simulink model "electro_mechanical_model"  (R2022a)
settings: Solver=VariableStepAuto  StartTime=0.0  StopTime=10000  RelTol=1e-3
values from neighbouring files (symbols this model uses):
  Ts = 5E-6    (= 5e-06)    [motor_variables.m]
undefined symbols (not defined in the file or in its folder): sigbuilder_block
libraries: fl_lib x42, nesl_utility x17, ee_lib x5, sdl_lib x2
settings Model: Creator=OADEBAJO  LastModifiedBy=oadebajo

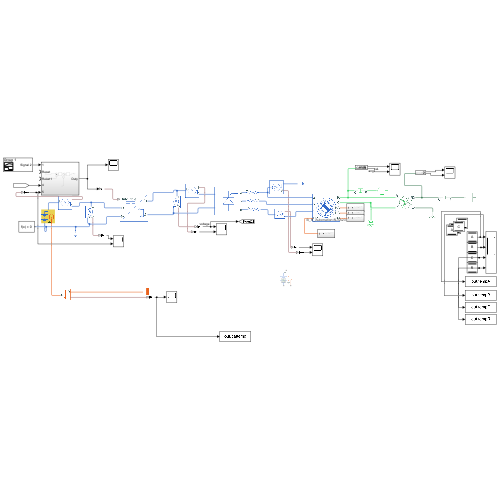
[thumbnail: Simulink's stored preview of the top-level diagram]
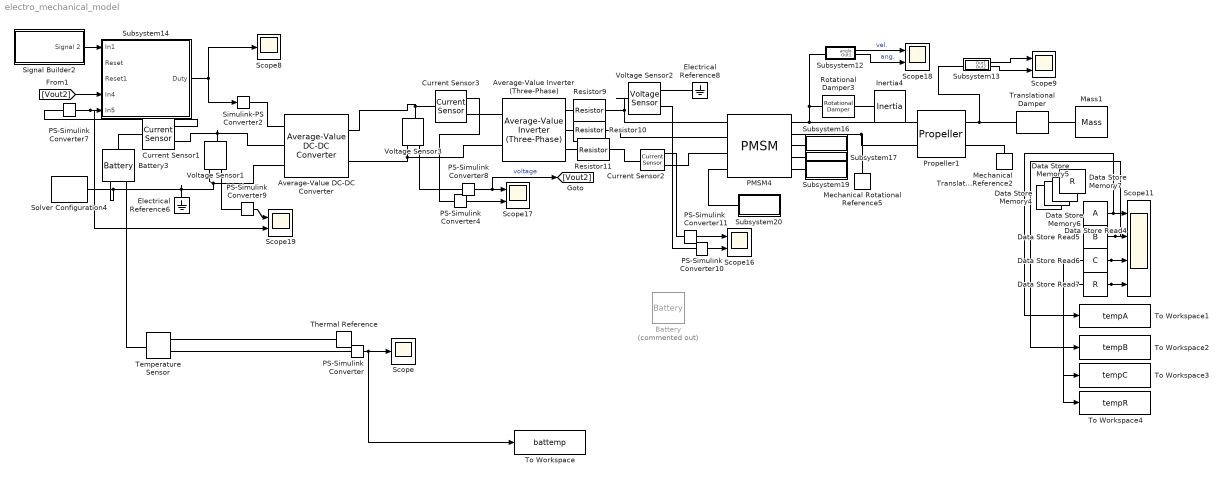
== system electro_mechanical_model ==
  Average-Value Inverter (Three-Phase) : ee_lib/Semiconductors & Converters/Converters/Average-Value Inverter (Three-Phase)  port_option=ee.enum.threePhasePort.expanded  FRated=60 Hz  PhaseShift=60 deg  voltage_ratio=sqrt(6) / pi  Pfixed=1e3 W  v_on=100 V  v_off=75 V
      settings: SourceProductBaseCode=PS  InternalSimscapePortConfiguration="{\"Bottom\":[],\"Left\":[{\"id\":\"p\",\"label\":\"+\",\"type\":\"foundation.electrical.electrical\"},{\"id\":\"n\",\"label\":\"-\",\"type\":\"foundation.electrical.electrical\"}],\"Right\":[{\"id\":\"a\",\"label\":\"a\",\"type\":\"foundation.electrical.electrical\"},{\"id\":\"b\",\"label\":\"b\",\"type\":\"foundation.electrical.electrical\"},{\"id\":\"c\",\"label\":\"c\",\"type\":\"foundation.electrical.electrical\"}],\"Top\":[]}"
  Average-Value DC-DC Converter : ee_lib/Semiconductors & Converters/Converters/Average-Value DC-DC Converter  control_option=ee.enum.converters.controlinput.dutycycle  converter_type=ee.enum.converters.dcdctype.buckboost  efficiency_option=ee.enum.converters.efficiency.constant  efficiency_fixed=100  i_vec=[0, 2, 5] A  efficiency_vec=[90, 95, 98]
      settings: SourceProductBaseCode=PS  InternalSimscapePortConfiguration="{\"Bottom\":[],\"Left\":[{\"id\":\"DutyCycle\",\"label\":\"DutyCycle\",\"type\":\"input\"},{\"id\":\"p1\",\"label\":\"1+\",\"type\":\"foundation.electrical.electrical\"},{\"id\":\"n1\",\"label\":\"1-\",\"type\":\"foundation.electrical.electrical\"}],\"Right\":[{\"id\":\"p2\",\"label\":\"2+\",\"type\":\"foundation.electrical.electrical\"},{\"id\":\"n2\",\"label\":\"2-\",\"type\":\"foundation.electrical.electrical\"}],\"Top\":[]}"
  Battery : ee_lib/Sources/Battery  Commented=on  Vnom=300 V  prm_dir=ee.enum.batterybasic.prm_dir.disabled  R1_dis=2 Ohm  R1_ch=2 Ohm  R1=0.001 Ohm  prm_AH=ee.enum.batterybasic.prm_AH.infinite  AH=50 A*hr  V1=11.5 V  AH1=25 A*hr  prm_R2=ee.enum.batterybasic.prm_R2.disabled  R2=2000 Ohm  prm_dyn=ee.enum.batterybasic.prm_dyn.off  Rp1=0.005 Ohm  tau1=30 s  Rp2=0.005 Ohm  tau2=30 s  Rp3=0.005 Ohm  tau3=30 s  Rp4=0.005 Ohm  tau4=30 s  Rp5=0.005 Ohm  tau5=30 s  prm_fade=ee.enum.batterybasic.prm_fade.disabled  N_fade=100  AH_fade=45 A*hr  R1_fade=2.02 Ohm  R1_ch_fade=2.02 Ohm  V1_fade=10.35 V  prm_age=ee.enum.batterybasic.prm_age.disabled  prm_age_OCV=ee.enum.batterybasic.prm_age_OCV.OCV  OCV_age=0.9  SOC_age=60  delta_time_age_vec=[0] d  temperature_age_vec=[273] K  OCV_scaling_age=2.2134e6  OCV_offset_age=1.632e6  temp_exp_age=0.515833569 V  t_exp_age=0.75  i_specify=off  i_priority=None  i=0 A  i_nominal_specify=off  i_nominal_unit=A  i_nominal_value=1  v_specify=off  v_priority=None  v=0 V  v_nominal_specify=off  v_nominal_unit=V  v_nominal_value=1  charge_specify=off  charge_priority=High  charge=50 A*hr  charge_nominal_specify=off  charge_nominal_unit=A*hr  charge_nominal_value=1  num_cycles_specify=off  num_cycles_priority=High  num_cycles=0  num_cycles_nominal_specify=off  num_cycles_nominal_unit=1  num_cycles_nominal_value=1  Tmeas=298.15 K  Tmeas_age=298.15 K  Vnom_T2=12 V  R1_T2=2.2 Ohm  R1_T2_dis=2.2 Ohm  R1_T2_ch=2.2 Ohm  V1_T2=11.4 V  R2_T2=2200 Ohm  Rp1_T2=0.005 Ohm  tau1_T2=30 s  Rp2_T2=0.005 Ohm  tau2_T2=30 s  Rp3_T2=0.005 Ohm  tau3_T2=30 s  Rp4_T2=0.005 Ohm  tau4_T2=30 s  Rp5_T2=0.005 Ohm  tau5_T2=30 s  Tmeas2=273.15 K  thermal_mass=30000 J/K  temperature_specify=off  temperature_priority=High  temperature=298.15 K  temperature_nominal_specify=off  temperature_nominal_unit=K  temperature_nominal_value=1
      settings: InternalSimscapePortConfiguration="{\"Bottom\":[],\"Left\":[{\"id\":\"p\",\"label\":\"+\",\"type\":\"foundation.electrical.electrical\"}],\"Right\":[{\"id\":\"n\",\"label\":\"-\",\"type\":\"foundation.electrical.electrical\"},{\"id\":\"H\",\"label\":\"H\",\"type\":\"foundation.thermal.thermal\"}],\"Top\":[]}"
  Battery3 : ee_lib/Sources/Battery  Vnom=300 V  prm_dir=ee.enum.batterybasic.prm_dir.disabled  R1_dis=2 Ohm  R1_ch=2 Ohm  R1=0.001 Ohm  prm_AH=ee.enum.batterybasic.prm_AH.infinite  AH=50 A*hr  V1=11.5 V  AH1=25 A*hr  prm_R2=ee.enum.batterybasic.prm_R2.disabled  R2=2000 Ohm  prm_dyn=ee.enum.batterybasic.prm_dyn.off  Rp1=0.005 Ohm  tau1=30 s  Rp2=0.005 Ohm  tau2=30 s  Rp3=0.005 Ohm  tau3=30 s  Rp4=0.005 Ohm  tau4=30 s  Rp5=0.005 Ohm  tau5=30 s  prm_fade=ee.enum.batterybasic.prm_fade.disabled  N_fade=100  AH_fade=45 A*hr  R1_fade=2.02 Ohm  R1_ch_fade=2.02 Ohm  V1_fade=10.35 V  prm_age=ee.enum.batterybasic.prm_age.disabled  prm_age_OCV=ee.enum.batterybasic.prm_age_OCV.OCV  OCV_age=0.9  SOC_age=60  delta_time_age_vec=[0] d  temperature_age_vec=[273] K  OCV_scaling_age=2.2134e6  OCV_offset_age=1.632e6  temp_exp_age=0.515833569 V  t_exp_age=0.75  i_specify=off  i_priority=None  i=0 A  i_nominal_specify=off  i_nominal_unit=A  i_nominal_value=1  v_specify=off  v_priority=None  v=0 V  v_nominal_specify=off  v_nominal_unit=V  v_nominal_value=1  charge_specify=off  charge_priority=High  charge=50 A*hr  charge_nominal_specify=off  charge_nominal_unit=A*hr  charge_nominal_value=1  num_cycles_specify=off  num_cycles_priority=High  num_cycles=0  num_cycles_nominal_specify=off  num_cycles_nominal_unit=1  num_cycles_nominal_value=1  Tmeas=298.15 K  Tmeas_age=298.15 K  Vnom_T2=300 V  R1_T2=0.01 Ohm  R1_T2_dis=2.2 Ohm  R1_T2_ch=2.2 Ohm  V1_T2=11.4 V  R2_T2=2200 Ohm  Rp1_T2=0.005 Ohm  tau1_T2=30 s  Rp2_T2=0.005 Ohm  tau2_T2=30 s  Rp3_T2=0.005 Ohm  tau3_T2=30 s  Rp4_T2=0.005 Ohm  tau4_T2=30 s  Rp5_T2=0.005 Ohm  tau5_T2=30 s  Tmeas2=273.15 K  thermal_mass=30000 J/K  temperature_specify=off  temperature_priority=High  temperature=298.15 K  temperature_nominal_specify=off  temperature_nominal_unit=K  temperature_nominal_value=1
      settings: InternalSimscapePortConfiguration="{\"Bottom\":[],\"Left\":[{\"id\":\"p\",\"label\":\"+\",\"type\":\"foundation.electrical.electrical\"}],\"Right\":[{\"id\":\"n\",\"label\":\"-\",\"type\":\"foundation.electrical.electrical\"},{\"id\":\"H\",\"label\":\"H\",\"type\":\"foundation.thermal.thermal\"}],\"Top\":[]}"
  Current Sensor1 : fl_lib/Electrical/Electrical Sensors/Current Sensor
      settings: SourceProductBaseCode=PW,SS,VE
  Current Sensor2 : fl_lib/Electrical/Electrical Sensors/Current Sensor
      settings: SourceProductBaseCode=PW,SS,VE
  Current Sensor3 : fl_lib/Electrical/Electrical Sensors/Current Sensor
      settings: SourceProductBaseCode=PW,SS,VE
  Data Store Memory4 : DataStoreMemory  WriteAfterWriteMsg=warning  ShowAdditionalParam=off
  Data Store Memory5 : DataStoreMemory  DataStoreName=B  WriteAfterWriteMsg=warning  ShowAdditionalParam=off
  Data Store Memory6 : DataStoreMemory  DataStoreName=C  WriteAfterWriteMsg=warning  ShowAdditionalParam=off
  Data Store Memory7 : DataStoreMemory  DataStoreName=R  WriteAfterWriteMsg=warning  ShowAdditionalParam=off
  Data Store Read4 : DataStoreRead  IndexOptions=Index vector (dialog)  Indices=1  OutputSizes=1
  Data Store Read5 : DataStoreRead  DataStoreName=B  IndexOptions=Index vector (dialog)  Indices=1  OutputSizes=1
  Data Store Read6 : DataStoreRead  DataStoreName=C  IndexOptions=Index vector (dialog)  Indices=1  OutputSizes=1
  Data Store Read7 : DataStoreRead  DataStoreName=R  IndexOptions=Index vector (dialog)  Indices=1  OutputSizes=1
  Electrical Reference6 : fl_lib/Electrical/Electrical Elements/Electrical Reference
      settings: SourceProductBaseCode=PW,SS,VE
  Electrical Reference8 : fl_lib/Electrical/Electrical Elements/Electrical Reference
      settings: SourceProductBaseCode=PW,SS,VE
  Inertia4 : fl_lib/Mechanical/Rotational Elements/Inertia  inertia=0.01 kg*m^2  num_ports=foundation.enum.numPorts2.one  w_specify=off  w_priority=High  w=0 rad/s  w_nominal_specify=off  w_nominal_unit=rad/s  w_nominal_value=1  t_specify=off  t_priority=None  t=0 N*m  t_nominal_specify=off  t_nominal_unit=N*m  t_nominal_value=1
      settings: SourceProductBaseCode=PW,SS,VE
  Mass1 : fl_lib/Mechanical/Translational Elements/Mass  mass=1 kg  num_ports=foundation.enum.numPorts2.one  v_specify=off  v_priority=High  v=0 m/s  v_nominal_specify=off  v_nominal_unit=m/s  v_nominal_value=1  f_specify=off  f_priority=None  f=0 N  f_nominal_specify=off  f_nominal_unit=N  f_nominal_value=1
      settings: SourceProductBaseCode=PW,SS,VE
  Mechanical Rotational Reference5 : fl_lib/Mechanical/Rotational Elements/Mechanical Rotational Reference
      settings: SourceProductBaseCode=PW,SS,VE
  Mechanical Translational Reference2 : fl_lib/Mechanical/Translational Elements/Mechanical Translational Reference
      settings: SourceProductBaseCode=PW,SS,VE
  PMSM4 : ee_lib/Electromechanical/Permanent Magnet/PMSM  Tag={'toolbox/physmod/elec/library/m/ee_lib_parts';'Electromechanical/Permanent_Magnet/PMSM/B_R_Automation/x8LSA23.xml'}  port_option=ee.enum.threePhasePort.expanded  winding_type=ee.enum.statorconnection.wye  machine_param=ee.enum.pmsm.parameterization.constant  nPolePairs=2  pmflux_param=ee.enum.pmflux.fluxlinkage  pm_flux_linkage=0.171455326591285 Wb  torque_constant=0.342910653182571 N*m/A  back_emf_constant=0.342910653182571 V/(rad/s)  stator_param=ee.enum.statorparam.LdLqL0  Ld=0.0825 H  Lq=0.0825 H  idVec=[-200 0 200] % Parameter not set A  iqVec=[-200 0 200] % Parameter not set A  LdMatrix=[0.0002 0.0002 0.0002;0.0002 0.0002 0.0002;0.0002 0.0002 0.0002] % Parameter not set H  LqMatrix=[0.0002 0.0002 0.0002;0.0002 0.0002 0.0002;0.0002 0.0002 0.0002] % Parameter not set H  PmMatrix=[0.1 0.1 0.1;0.1 0.1 0.1;0.1 0.1 0.1] Wb  ktMatrix=[0.18 0.18 0.18;0.18 0.18 0.18;0.18 0.18 0.18] N*m/A  keMatrix=[0.18 0.18 0.18;0.18 0.18 0.18;0.18 0.18 0.18] % Parameter not set V/(rad/s)  L0=[] % Parameter not set H  Ls=0.0002 H  Lm=-2e-05 H  Ms=2e-05 H  Rs=84 Ohm  zero_sequence=ee.enum.park.zerosequence.exclude  axes_param=ee.enum.rotorangle.daxis  loss_param=ee.enum.ironloss.none  losses_oc=[0 0 0] % Parameter not set W  losses_sc=[0 0 0] % Parameter not set W  f_losses=60 % Parameter not set Hz  Isc_losses=95 % Parameter not set A  J=7e-06 kg*m^2  lam=0 % Parameter not set N*m/(rad/s)  i_d_specify=off  i_d_priority=None  i_d=0 A  i_d_nominal_specify=off  i_d_nominal_unit=A  i_d_nominal_value=1  i_q_specify=off  i_q_priority=None  i_q=0 A  i_q_nominal_specify=off  i_q_nominal_unit=A  i_q_nominal_value=1  torque_specify=off  torque_priority=None  torque=0 N*m  torque_nominal_specify=off  torque_nominal_unit=N*m  torque_nominal_value=1  angular_velocity_specify=off  angular_velocity_priority=High  angular_velocity=0 rpm  angular_velocity_nominal_specify=off  angular_velocity_nominal_unit=rpm  angular_velocity_nominal_value=1  angular_position_specify=off  angular_position_priority=High  angular_position=0 deg  angular_position_nominal_specify=off  angular_position_nominal_unit=deg  angular_position_nominal_value=1  alpha=0.00393 % Parameter not set 1/K  alpha_flux=-0.001 % Parameter not set 1/K  Tmeas=298.15 % Parameter not set K  stator_thermal_mass=100 % Parameter not set J/K  rotor_thermal_mass=200 % Parameter not set J/K  Rm_percent_rotor=90  Rd_percent_rotor=30  temperatureA_specify=on  temperatureA_priority=None  temperatureA=25 degC  temperatureA_nominal_specify=off  temperatureA_nominal_unit=degC  temperatureA_nominal_value=1  temperatureB_specify=on  temperatureB_priority=None  temperatureB=25 degC  temperatureB_nominal_specify=off  temperatureB_nominal_unit=degC  temperatureB_nominal_value=1  temperatureC_specify=on  temperatureC_priority=None  temperatureC=25 degC  temperatureC_nominal_specify=off  temperatureC_nominal_unit=degC  temperatureC_nominal_value=1  temperatureR_specify=on  temperatureR_priority=None  temperatureR=25 degC  temperatureR_nominal_specify=off  temperatureR_nominal_unit=degC  temperatureR_nominal_value=1
      settings: AttributesFormatString=B_R_Automation:8LSA23  InternalSimscapePortConfiguration="{\"Bottom\":[],\"Left\":[{\"id\":\"a\",\"label\":\"a\",\"type\":\"foundation.electrical.electrical\"},{\"id\":\"b\",\"label\":\"b\",\"type\":\"foundation.electrical.electrical\"},{\"id\":\"c\",\"label\":\"c\",\"type\":\"foundation.electrical.electrical\"},{\"id\":\"HR\",\"label\":\"HR\",\"type\":\"foundation.thermal.thermal\"}],\"Right\":[{\"id\":\"R\",\"label\":\"R\",\"type\":\"foundation.mechanical.rotational.rotational\"},{\"id\":\"C\",\"label\":\"C\",\"type\":\"foundation.mechanical.rotational.rotational\"},{\"id\":\"HA\",\"label\":\"HA\",\"type\":\"foundation.thermal.thermal\"},{\"id\":\"HB\",\"label\":\"HB\",\"type\":\"foundation.thermal.thermal\"},{\"id\":\"HC\",\"label\":\"HC\",\"type\":\"foundation.thermal.thermal\"}],\"Top\":[]}"
  PS-Simulink Converter{,4,10..11} (4 alike) : nesl_utility/PS-Simulink Converter  PhysicalDomain=network_engine_domain  SubClassName=ps_output  LeftPortType=input  RightPortType=output  PseudoPeriodic=off  Frequencies=[]  VectorFormat=inherit  Unit=inherit  AffineConversion=off
      settings: SourceProductBaseCode=SS,PW,VE
  PS-Simulink Converter7 : nesl_utility/PS-Simulink Converter  PhysicalDomain=network_engine_domain  SubClassName=ps_output  LeftPortType=input  RightPortType=output  PseudoPeriodic=off  Frequencies=[]  VectorFormat=1-D array  Unit=A  AffineConversion=off
      settings: SourceProductBaseCode=SS,PW,VE
  PS-Simulink Converter8 : nesl_utility/PS-Simulink Converter  PhysicalDomain=network_engine_domain  SubClassName=ps_output  LeftPortType=input  RightPortType=output  PseudoPeriodic=off  Frequencies=[]  VectorFormat=1-D array  Unit=V  AffineConversion=off
      settings: SourceProductBaseCode=SS,PW,VE
  PS-Simulink Converter9 : nesl_utility/PS-Simulink Converter  PhysicalDomain=network_engine_domain  SubClassName=ps_output  LeftPortType=input  RightPortType=output  PseudoPeriodic=off  Frequencies=[]  VectorFormat=1-D array  Unit=V  AffineConversion=off
      settings: SourceProductBaseCode=SS,PW,VE
  Propeller1 : sdl_lib/Engines & Motors/Propeller  parameterization=sdl.enum.PropellerParameterization.Constant  pitch_type=foundation.enum.constant_controlled.constant  D=0.2 m  kt_const=0.25  kq_const=0.05  kt_poly_fixed=[.063, -.19, -.25, .37]  kq_poly_fixed=[.0043, -.021, -.03, .05]  pitch_ratio_TLU=[-.5, .5, .7, .9, 1.1, 1.4]  kt_poly_TLU=[.04, -.1, -.24, .12; .118, -.24, -.24, .19; .082, -.21, -.25, .28; .063, -.19, -.25, .37; .055, -.17, -.25, .45; .064, -.21, -.19, .55]  kq_poly_TLU=[.02, -.06, -.02, .02; .04, -.034, -.016, .018; .0076, -.02, -.023, .031; .0043, -.021, -.03, .05; .0047, -.024, -.036, .073; .0045, -.025, -.044, .11]  J_tab_TLU=[0, .3, .5, .7, .9, 1.2, 1.5]  kt_tab_fixed=[.37, .28, .21, .12, .033, -.098, -.23]  kq_tab_fixed=[.049, .039, .03, .02, .0096, -.0093, -.028]  kt_tab_TLU=[.12, .04, -.02, -.083, -.15, -.24, -.33; .19, .1, .029, -.047, -.12, -.23, -.35; .28, .19, .12, .032, -.054, -.18, -.31; .37, .28, .21, .12, .033, -.098, -.23; .45, .36, .29, .21, .13, -.0057, -.16; .54, .47, .41, .33, .25, .13, .0029]  kq_tab_TLU=[.02, .0091, -.0025, -.017, -.032, -.056, -.078; .017, .011, .006, .0009, -.0041, -.012, -.019; .03, .022, .015, .0074, -.0008, -.013, -.026; .049, .039, .03, .02, .0096, -.0093, -.028; .072, .06, .05, .038, .025, .0042, -.015; .11, .097, .085, .071, .057, .033, .0065]  interp_method=simscape.enum.interpolation.linear  extrap_method=simscape.enum.extrapolation.linear  density_spec=foundation.enum.constant_variable.constant  rho=1000 kg/m^3  translational_ports=sdl.enum.ConnectionType.Conserving  wake_fraction=0.2  efficiency_sensor=simscape.enum.onoff.off  n_thr=0.001 Hz  k_thr=0.001  operation_check=simscape.enum.assert.action.warn  w_specify=off  w_priority=None  w=0 rad/s  w_nominal_specify=off  w_nominal_unit=rad/s  w_nominal_value=1  Q_specify=off  Q_priority=None  Q=0 N*m  Q_nominal_specify=off  Q_nominal_unit=N*m  Q_nominal_value=1  v_specify=off  v_priority=None  v=0 m/s  v_nominal_specify=off  v_nominal_unit=m/s  v_nominal_value=1  thrust_specify=off  thrust_priority=None  thrust=0 N  thrust_nominal_specify=off  thrust_nominal_unit=N  thrust_nominal_value=1
      settings: SourceProductBaseCode=LD  InternalSimscapePortConfiguration="{\"Bottom\":[],\"Left\":[{\"id\":\"R1\",\"label\":\"R1\",\"type\":\"foundation.mechanical.rotational.rotational\"},{\"id\":\"C1\",\"label\":\"C1\",\"type\":\"foundation.mechanical.rotational.rotational\"}],\"Right\":[{\"id\":\"R2\",\"label\":\"R2\",\"type\":\"foundation.mechanical.translational.translational\"},{\"id\":\"C2\",\"label\":\"C2\",\"type\":\"foundation.mechanical.translational.translational\"}],\"Top\":[]}"
  Resistor10 : fl_lib/Electrical/Electrical Elements/Resistor  R=10 Ohm  i_specify=off  i_priority=None  i=0 A  i_nominal_specify=off  i_nominal_unit=A  i_nominal_value=1  v_specify=off  v_priority=None  v=0 V  v_nominal_specify=off  v_nominal_unit=V  v_nominal_value=1
      settings: SourceProductBaseCode=PW,SS,VE
  Resistor11 : fl_lib/Electrical/Electrical Elements/Resistor  R=10 Ohm  i_specify=off  i_priority=None  i=0 A  i_nominal_specify=off  i_nominal_unit=A  i_nominal_value=1  v_specify=off  v_priority=None  v=0 V  v_nominal_specify=off  v_nominal_unit=V  v_nominal_value=1
      settings: SourceProductBaseCode=PW,SS,VE
  Resistor9 : fl_lib/Electrical/Electrical Elements/Resistor  R=10 Ohm  i_specify=off  i_priority=None  i=0 A  i_nominal_specify=off  i_nominal_unit=A  i_nominal_value=1  v_specify=off  v_priority=None  v=0 V  v_nominal_specify=off  v_nominal_unit=V  v_nominal_value=1
      settings: SourceProductBaseCode=PW,SS,VE
  Rotational Damper3 : sdl_lib/Couplings & Drives/Springs & Dampers/Rotational Damper  D=1e-3 N*m*s/rad  enable_faults=simscape.enum.onoff.off  b_fault=100 N*m*s/rad  temporal_fault=simscape.enum.onoff.off  fault_time=5 s  shock_fault=simscape.enum.onoff.off  acceleration_limit=100 rad/s^2  shock_limit=1  report_fault=simscape.enum.assert.action.none  thermal_port=simscape.enum.thermaleffects.omit  thermal_mass=50 kJ/K  temperature_specify=off  temperature_priority=High  temperature=300 K  temperature_nominal_specify=off  temperature_nominal_unit=K  temperature_nominal_value=1
      settings: SourceProductBaseCode=LD
  Scope : Scope
  Scope11 : Scope  NumInputPorts=4
  Scope{9,16..19} (5 alike) : Scope  NumInputPorts=2
  Scope8 : Scope
  Signal Builder2 : Subsystem  Tag=STV Subsys  LoadFcn=sigbuilder_block('load');  StartFcn=sigbuilder_block('start');  StopFcn=sigbuilder_block('stop');  ClipboardFcn=sigbuilder_block('clipboard');  mask(Sigbuilder block){tuvar=[0:10]}
      mask help: Simulink:masks:SigbuilderBlock_MD
      mask init:
      | if ~strcmp(get_param(bdroot(gcbh),'SimulationStatus'),'stopped') tuvar = sigbuilder_block('maskInit'); end
      settings: CopyFcn=sigbuilder_block('copy');  DeleteFcn=sigbuilder_block('delete');  ModelCloseFcn=sigbuilder_block('modelClose');  PreSaveFcn=sigbuilder_block('preSave');  PauseFcn=sigbuilder_block('pause');  ContinueFcn=sigbuilder_block('continue');  NameChangeFcn=sigbuilder_block('namechange');  OpenFcn=sigbuilder_block('open',[4.875 4.875 836.25 501.75 ]);  CloseFcn=sigbuilder_block('close');
      mask Display: plot(0, 0, 100, 100,[2, 2, 32, 32, 2], [68, 8, 8, 68, 68],[32, 2], [38, 38], [32, 19, 2],[53, 60, 44], [32, 17, 17, 2],[16, 16, 31, 31]);txt = getActiveGroup(gcbh);text(2, 100, txt,'verticalAlignment', 'top');
  Simulink-PS Converter2 : nesl_utility/Simulink-PS Converter  PhysicalDomain=network_engine_domain  SubClassName=ps_input  LeftPortType=input  RightPortType=output  PseudoPeriodic=off  Frequencies=[]  NoiseDistribution=none  NoiseParameters=[]  Unit=1  AffineConversion=off  FilteringAndDerivatives=provide  SimscapeFilterOrder=1  InputFilterTimeConstant=0.001  UdotUserProvided=0
      settings: SourceProductBaseCode=SS,PW,VE
  Solver Configuration4 : nesl_utility/Solver Configuration  PhysicalDomain=network_engine_domain  SubClassName=solver  LeftPortType=input  RightPortType=generic  Tones=[]  Harmonics=[]  SimulateNoise=off  Profile=off  UseLocalSampling=off  EnableSwitchedLinearOptims=on  FrequencyDomain=off  UseCCode=off  RelTol=0.001  AbsTol=1e-06  MinStep=1e-09  ToWorkspace=off  RevertToSquareIcSolve=off  NumHomotopyIterations=100  PhasorMode=off  PhasorModeNumHarmonics=1  IndexReductionMethod=DerivativeReplacement  DoDC=off  ResidualTolerance=1e-3  UseLocalSolver=on  LocalSolverChoice=NE_BACKWARD_EULER_ADVANCER  LocalSolverSampleTime=1e-4  DoFixedCost=on  MaxNonlinIter=3  MaxModeIter=2  ComputeImpulses=off  ImpulseIterations=2  LinearAlgebra=auto  LinearAlgebraNumThread=0  EquationFormulation=NE_TIME_EF  DelaysMemoryBudget=1024  AutomaticFiltering=off  FilteringTimeConstant=0.001  PartitionStorageMethod=AS_NEEDED  PartitionMemoryBudget=1024  PartitionMethod=FAST
      settings: SourceProductBaseCode=SS,PW,VE
  Subsystem12 : Subsystem
  Subsystem13 : Subsystem
  Subsystem14 : Subsystem
  Subsystem16 : Subsystem
  Subsystem17 : Subsystem
  Subsystem19 : Subsystem
  Subsystem20 : Subsystem
  Temperature Sensor : fl_lib/Thermal/Thermal Sensors/Temperature Sensor
      settings: SourceProductBaseCode=PW,SS,VE
  Thermal Reference : fl_lib/Thermal/Thermal Elements/Thermal Reference
      settings: SourceProductBaseCode=PW,SS,VE
  To Workspace : ToWorkspace  VariableName=battemp  SaveFormat=Timeseries  SampleTime=-1
  To Workspace1 : ToWorkspace  VariableName=tempA  SaveFormat=Timeseries  SampleTime=-1
  To Workspace2 : ToWorkspace  VariableName=tempB  SaveFormat=Timeseries  SampleTime=-1
  To Workspace3 : ToWorkspace  VariableName=tempC  SaveFormat=Timeseries  SampleTime=-1
  To Workspace4 : ToWorkspace  VariableName=tempR  SaveFormat=Timeseries  SampleTime=-1
  Translational Damper : fl_lib/Mechanical/Translational Elements/Translational Damper  D=100 N*s/m  v_specify=off  v_priority=None  v=0 m/s  v_nominal_specify=off  v_nominal_unit=m/s  v_nominal_value=1  f_specify=off  f_priority=None  f=0 N  f_nominal_specify=off  f_nominal_unit=N  f_nominal_value=1
      settings: SourceProductBaseCode=PW,SS,VE
  Voltage Sensor1 : fl_lib/Electrical/Electrical Sensors/Voltage Sensor
      settings: SourceProductBaseCode=PW,SS,VE
  Voltage Sensor2 : fl_lib/Electrical/Electrical Sensors/Voltage Sensor
      settings: SourceProductBaseCode=PW,SS,VE
  Voltage Sensor3 : fl_lib/Electrical/Electrical Sensors/Voltage Sensor
      settings: SourceProductBaseCode=PW,SS,VE
  wires:
  PS-Simulink Converter/1 -> To Workspace/1, Scope/1
  PS-Simulink Converter8/1 -> [Vout2], Scope17/1  "voltage"
  Subsystem12/2(Out1) -> Scope18/2  "ang."
  PS-Simulink Converter7/1 -> Scope19/2, Subsystem14/5(In5)
  Subsystem12/1(angle) -> Scope18/1  "vel."
  Subsystem13/1(Out1) -> Scope9/1
  Data Store Read5/1 -> To Workspace2/1, Scope11/2
  [Vout2] -> Subsystem14/4(In4)
  Signal Builder2/1(Signal 2) -> Subsystem14/1(In1)
  PS-Simulink Converter10/1 -> Scope16/2
  PS-Simulink Converter9/1 -> Scope19/1
  Data Store Read6/1 -> Scope11/3, To Workspace3/1
  Subsystem14/1(Duty) -> Simulink-PS Converter2/1, Scope8/1
  PS-Simulink Converter11/1 -> Scope16/1
  Data Store Read7/1 -> Scope11/4, To Workspace4/1
  Subsystem13/2(Out2) -> Scope9/2
  PS-Simulink Converter4/1 -> Scope17/2
  Data Store Read4/1 -> To Workspace1/1, Scope11/1
  connections:
  Average-Value DC-DC Converter/RConn2 -- Voltage Sensor3/RConn2 -- Average-Value Inverter (Three-Phase)/LConn2
  Resistor9/RConn1 -- PMSM4/LConn1 -- Voltage Sensor2/LConn1
  Propeller1/LConn1 -- PMSM4/RConn1 -- Rotational Damper3/RConn1 -- Subsystem12/LConn1
  Propeller1/RConn1 -- Subsystem13/LConn1 -- Translational Damper/RConn1
  Mechanical Rotational Reference5/LConn1 -- PMSM4/RConn2 -- Propeller1/LConn2
  Average-Value DC-DC Converter/LConn2 -- Voltage Sensor1/LConn1 -- Current Sensor1/RConn2
  Average-Value DC-DC Converter/RConn1 -- Voltage Sensor3/LConn1 -- Current Sensor3/LConn1
  Electrical Reference6/LConn1 -- Battery3/RConn1 -- Solver Configuration4/RConn1 -- Average-Value DC-DC Converter/LConn3 -- Voltage Sensor1/RConn2
  Voltage Sensor2/RConn2 -- Electrical Reference8/LConn1
  Thermal Reference/LConn1 -- Temperature Sensor/RConn1
  Current Sensor3/RConn2 -- Average-Value Inverter (Three-Phase)/LConn1
  PS-Simulink Converter/LConn1 -- Temperature Sensor/RConn2
  Subsystem17/LConn1 -- PMSM4/RConn4
  Battery3/RConn2 -- Temperature Sensor/LConn1
  Average-Value Inverter (Three-Phase)/RConn3 -- Resistor11/LConn1
  Subsystem20/LConn1 -- PMSM4/LConn4
  Resistor10/RConn1 -- PMSM4/LConn2
  PS-Simulink Converter7/LConn1 -- Current Sensor1/RConn1
  Current Sensor2/LConn1 -- Resistor11/RConn1
  Current Sensor2/RConn1 -- PS-Simulink Converter11/LConn1
  Average-Value Inverter (Three-Phase)/RConn2 -- Resistor10/LConn1
  Average-Value DC-DC Converter/LConn1 -- Simulink-PS Converter2/RConn1
  Battery3/LConn1 -- Current Sensor1/LConn1
  PS-Simulink Converter4/LConn1 -- Current Sensor3/RConn1
  Voltage Sensor1/RConn1 -- PS-Simulink Converter9/LConn1
  PS-Simulink Converter8/LConn1 -- Voltage Sensor3/RConn1
  Translational Damper/LConn1 -- Mass1/LConn1
  PMSM4/RConn5 -- Subsystem19/LConn1
  Propeller1/RConn2 -- Mechanical Translational Reference2/LConn1
  Current Sensor2/RConn2 -- PMSM4/LConn3
  Inertia4/LConn1 -- Rotational Damper3/LConn1
  Voltage Sensor2/RConn1 -- PS-Simulink Converter10/LConn1
  PMSM4/RConn3 -- Subsystem16/LConn1
  Average-Value Inverter (Three-Phase)/RConn1 -- Resistor9/LConn1

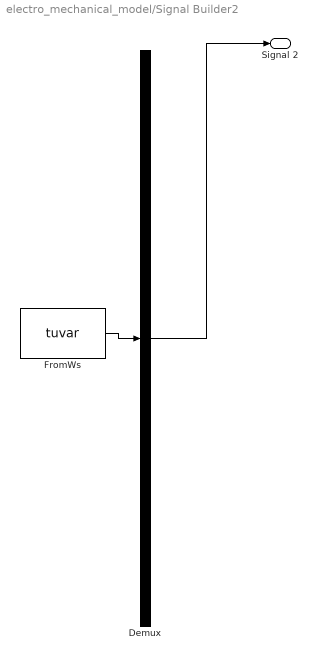
== system electro_mechanical_model/Signal Builder2 ==
  Demux : Demux  Tag=STV Demux  Outputs=1
      settings: DisplayOption=none
  FromWs : FromWorkspace  Tag=STV FromWs  VariableName=tuvar
      SigBuilderData=|
      | common.afterFinalStr = 'Extrapolate'
      | common.sampleTime = 0
      | dataSet.timeRange = [0 3600]
      | dataSet.name = 'Group 1'
      | sbobj.Groups.Name = 'Group 1'
      | sbobj.Groups.Signals.Name = 'Signal 2'
      | sbobj.Groups.Signals.XData = [0 4 4 1800 2500 2500 3600]
      | sbobj.Groups.Signals.YData = [270 270 315 315 317.5 340 350]
      | sbobj.Groups.TimeRange = [0 3600]
  Signal 2 : Outport  Tag=STV Outport
  wires:
  FromWs/1 -> Demux/1
  Demux/1 -> Signal 2/1

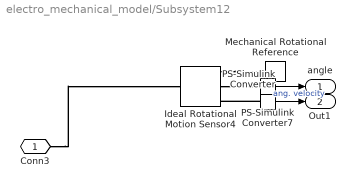
== system electro_mechanical_model/Subsystem12 ==
  Ideal Rotational Motion Sensor4 : fl_lib/Mechanical/Mechanical Sensors/Ideal Rotational Motion Sensor  wrap_angle=simscape.enum.onoff.off  offset=0 rad
      settings: SourceProductBaseCode=PW,SS,VE
  Mechanical Rotational Reference : fl_lib/Mechanical/Rotational Elements/Mechanical Rotational Reference
      settings: SourceProductBaseCode=PW,SS,VE
  PS-Simulink Converter : nesl_utility/PS-Simulink Converter  PhysicalDomain=network_engine_domain  SubClassName=ps_output  LeftPortType=input  RightPortType=output  PseudoPeriodic=off  Frequencies=[]  VectorFormat=inherit  Unit=inherit  AffineConversion=off
      settings: SourceProductBaseCode=SS,PW,VE
  PS-Simulink Converter7 : nesl_utility/PS-Simulink Converter  PhysicalDomain=network_engine_domain  SubClassName=ps_output  LeftPortType=input  RightPortType=output  PseudoPeriodic=off  Frequencies=[]  VectorFormat=inherit  Unit=inherit  AffineConversion=off
      settings: SourceProductBaseCode=SS,PW,VE
  Conn3 : PMIOPort  Side=Left
  angle : Outport
  Out1 : Outport  Port=2
  wires:
  PS-Simulink Converter7/1 -> angle/1  "ang. velocity"
  PS-Simulink Converter/1 -> Out1/1
  connections:
  Ideal Rotational Motion Sensor4/RConn2 -- PS-Simulink Converter7/LConn1
  PS-Simulink Converter/LConn1 -- Ideal Rotational Motion Sensor4/RConn3
  Conn3/RConn1 -- Ideal Rotational Motion Sensor4/LConn1
  Ideal Rotational Motion Sensor4/RConn1 -- Mechanical Rotational Reference/LConn1

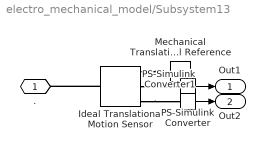
== system electro_mechanical_model/Subsystem13 ==
  Ideal Translational Motion Sensor : fl_lib/Mechanical/Mechanical Sensors/Ideal Translational Motion Sensor  offset=0 m
      settings: SourceProductBaseCode=PW,SS,VE
  Mechanical Translational Reference : fl_lib/Mechanical/Translational Elements/Mechanical Translational Reference
      settings: SourceProductBaseCode=PW,SS,VE
  PS-Simulink Converter : nesl_utility/PS-Simulink Converter  PhysicalDomain=network_engine_domain  SubClassName=ps_output  LeftPortType=input  RightPortType=output  PseudoPeriodic=off  Frequencies=[]  VectorFormat=inherit  Unit=inherit  AffineConversion=off
      settings: SourceProductBaseCode=SS,PW,VE
  PS-Simulink Converter1 : nesl_utility/PS-Simulink Converter  PhysicalDomain=network_engine_domain  SubClassName=ps_output  LeftPortType=input  RightPortType=output  PseudoPeriodic=off  Frequencies=[]  VectorFormat=inherit  Unit=inherit  AffineConversion=off
      settings: SourceProductBaseCode=SS,PW,VE
  . : PMIOPort  Side=Left
  Out1 : Outport
  Out2 : Outport  Port=2
  wires:
  PS-Simulink Converter/1 -> Out1/1
  PS-Simulink Converter1/1 -> Out2/1
  connections:
  Ideal Translational Motion Sensor/LConn1 -- ./RConn1
  Ideal Translational Motion Sensor/RConn2 -- PS-Simulink Converter/LConn1
  Ideal Translational Motion Sensor/RConn3 -- PS-Simulink Converter1/LConn1
  Ideal Translational Motion Sensor/RConn1 -- Mechanical Translational Reference/LConn1

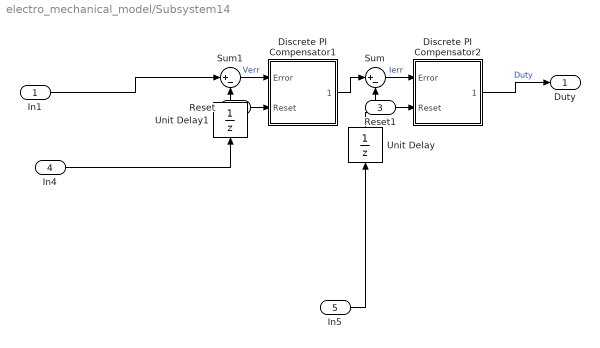
== system electro_mechanical_model/Subsystem14 ==
  In1 : Inport
  Reset : Inport  Port=2
  Reset1 : Inport  Port=3
  In4 : Inport  Port=4
  In5 : Inport  Port=5
  Discrete PI Compensator1 : Subsystem  mask{Kp=2.593/10000, Ki=1496.8*1, Ts_PI=Ts, UpSat=35, LowSat=-35, Initial_Condition=0}
      mask prompts: Kp "Kp Value"; Ki "Ki Value"; Ts_PI "Sample Time"; UpSat "Saturation Upper Limit"; LowSat "Saturation Lower Limit"; Initial_Condition "Initial Condition"
      mask DialogControl DescTextVar Prompt: %<Discrete PI Compensator using trapezoidal approximation for integration with saturation and back-clamping.>
  Discrete PI Compensator2 : Subsystem  mask{Kp=0.31/100, Ki=4534.18/100, Ts_PI=Ts, UpSat=0.9, LowSat=0, Initial_Condition=0}
      mask prompts: Kp "Kp Value"; Ki "Ki Value"; Ts_PI "Sample Time"; UpSat "Saturation Upper Limit"; LowSat "Saturation Lower Limit"; Initial_Condition "Initial Condition"
      mask DialogControl DescTextVar Prompt: %<Discrete PI Compensator using trapezoidal approximation for integration with saturation and back-clamping.>
  Sum : Sum  Inputs=|+-
  Sum1 : Sum  Inputs=|+-
  Unit Delay : UnitDelay  SampleTime=-1  HasFrameUpgradeWarning=on
  Unit Delay1 : UnitDelay  SampleTime=-1  HasFrameUpgradeWarning=on
  Duty : Outport
  wires:
  Sum/1 -> Discrete PI Compensator2/1(Error)  "Ierr"
  Unit Delay/1 -> Sum/2
  Unit Delay1/1 -> Sum1/2
  Discrete PI Compensator2/1(Signal Out) -> Duty/1  "Duty"
  Sum1/1 -> Discrete PI Compensator1/1(Error)  "Verr"
  Discrete PI Compensator1/1(Signal Out) -> Sum/1
  In1/1 -> Sum1/1
  In4/1 -> Unit Delay1/1
  In5/1 -> Unit Delay/1
  Reset1/1 -> Discrete PI Compensator2/2(Reset)
  Reset/1 -> Discrete PI Compensator1/2(Reset)

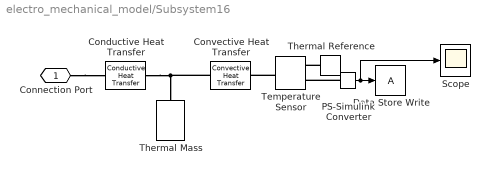
== system electro_mechanical_model/Subsystem16 ==
  Conductive Heat Transfer : fl_lib/Thermal/Thermal Elements/Conductive Heat Transfer  area=1e-4 m^2  thickness=0.1 m  th_cond=401 W/(K*m)  T_specify=off  T_priority=None  T=0 K  T_nominal_specify=off  T_nominal_unit=K  T_nominal_value=1  Q_specify=off  Q_priority=None  Q=0 W  Q_nominal_specify=off  Q_nominal_unit=W  Q_nominal_value=1
      settings: SourceProductBaseCode=PW,SS,VE
  Convective Heat Transfer : fl_lib/Thermal/Thermal Elements/Convective Heat Transfer  area=1e-4 m^2  heat_tr_coeff=20 W/(K*m^2)  T_specify=off  T_priority=None  T=0 K  T_nominal_specify=off  T_nominal_unit=K  T_nominal_value=1  Q_specify=off  Q_priority=None  Q=0 W  Q_nominal_specify=off  Q_nominal_unit=W  Q_nominal_value=1
      settings: SourceProductBaseCode=PW,SS,VE
  Data Store Write : DataStoreWrite  IndexOptions=Index vector (dialog)  Indices=1  OutputSizes=1
  PS-Simulink Converter : nesl_utility/PS-Simulink Converter  PhysicalDomain=network_engine_domain  SubClassName=ps_output  LeftPortType=input  RightPortType=output  PseudoPeriodic=off  Frequencies=[]  VectorFormat=inherit  Unit=inherit  AffineConversion=off
      settings: SourceProductBaseCode=SS,PW,VE
  Scope : Scope
  Temperature Sensor : fl_lib/Thermal/Thermal Sensors/Temperature Sensor
      settings: SourceProductBaseCode=PW,SS,VE
  Thermal Mass : fl_lib/Thermal/Thermal Elements/Thermal Mass  mass=1 kg  sp_heat=447 J/(K*kg)  T_specify=off  T_priority=High  T=300 K  T_nominal_specify=off  T_nominal_unit=K  T_nominal_value=1  Q_specify=off  Q_priority=None  Q=0 W  Q_nominal_specify=off  Q_nominal_unit=W  Q_nominal_value=1
      settings: SourceProductBaseCode=PW,SS,VE
  Thermal Reference : fl_lib/Thermal/Thermal Elements/Thermal Reference
      settings: SourceProductBaseCode=PW,SS,VE
  Connection Port : PMIOPort  Side=Left
  wires:
  PS-Simulink Converter/1 -> Scope/1, Data Store Write/1
  connections:
  Connection Port/RConn1 -- Conductive Heat Transfer/LConn1
  Conductive Heat Transfer/RConn1 -- Convective Heat Transfer/LConn1 -- Thermal Mass/LConn1
  Temperature Sensor/LConn1 -- Convective Heat Transfer/RConn1
  Thermal Reference/LConn1 -- Temperature Sensor/RConn1
  PS-Simulink Converter/LConn1 -- Temperature Sensor/RConn2

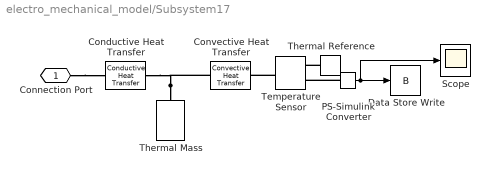
== system electro_mechanical_model/Subsystem17 ==
  Conductive Heat Transfer : fl_lib/Thermal/Thermal Elements/Conductive Heat Transfer  area=1e-4 m^2  thickness=0.1 m  th_cond=401 W/(K*m)  T_specify=off  T_priority=None  T=0 K  T_nominal_specify=off  T_nominal_unit=K  T_nominal_value=1  Q_specify=off  Q_priority=None  Q=0 W  Q_nominal_specify=off  Q_nominal_unit=W  Q_nominal_value=1
      settings: SourceProductBaseCode=PW,SS,VE
  Convective Heat Transfer : fl_lib/Thermal/Thermal Elements/Convective Heat Transfer  area=1e-4 m^2  heat_tr_coeff=20 W/(K*m^2)  T_specify=off  T_priority=None  T=0 K  T_nominal_specify=off  T_nominal_unit=K  T_nominal_value=1  Q_specify=off  Q_priority=None  Q=0 W  Q_nominal_specify=off  Q_nominal_unit=W  Q_nominal_value=1
      settings: SourceProductBaseCode=PW,SS,VE
  Data Store Write : DataStoreWrite  DataStoreName=B  IndexOptions=Index vector (dialog)  Indices=1  OutputSizes=1
  PS-Simulink Converter : nesl_utility/PS-Simulink Converter  PhysicalDomain=network_engine_domain  SubClassName=ps_output  LeftPortType=input  RightPortType=output  PseudoPeriodic=off  Frequencies=[]  VectorFormat=inherit  Unit=inherit  AffineConversion=off
      settings: SourceProductBaseCode=SS,PW,VE
  Scope : Scope
  Temperature Sensor : fl_lib/Thermal/Thermal Sensors/Temperature Sensor
      settings: SourceProductBaseCode=PW,SS,VE
  Thermal Mass : fl_lib/Thermal/Thermal Elements/Thermal Mass  mass=1 kg  sp_heat=447 J/(K*kg)  T_specify=off  T_priority=High  T=300 K  T_nominal_specify=off  T_nominal_unit=K  T_nominal_value=1  Q_specify=off  Q_priority=None  Q=0 W  Q_nominal_specify=off  Q_nominal_unit=W  Q_nominal_value=1
      settings: SourceProductBaseCode=PW,SS,VE
  Thermal Reference : fl_lib/Thermal/Thermal Elements/Thermal Reference
      settings: SourceProductBaseCode=PW,SS,VE
  Connection Port : PMIOPort  Side=Left
  wires:
  PS-Simulink Converter/1 -> Data Store Write/1, Scope/1
  connections:
  Connection Port/RConn1 -- Conductive Heat Transfer/LConn1
  Thermal Mass/LConn1 -- Conductive Heat Transfer/RConn1 -- Convective Heat Transfer/LConn1
  Temperature Sensor/LConn1 -- Convective Heat Transfer/RConn1
  Thermal Reference/LConn1 -- Temperature Sensor/RConn1
  PS-Simulink Converter/LConn1 -- Temperature Sensor/RConn2

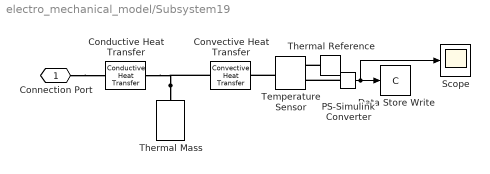
== system electro_mechanical_model/Subsystem19 ==
  Conductive Heat Transfer : fl_lib/Thermal/Thermal Elements/Conductive Heat Transfer  area=1e-4 m^2  thickness=0.1 m  th_cond=401 W/(K*m)  T_specify=off  T_priority=None  T=0 K  T_nominal_specify=off  T_nominal_unit=K  T_nominal_value=1  Q_specify=off  Q_priority=None  Q=0 W  Q_nominal_specify=off  Q_nominal_unit=W  Q_nominal_value=1
      settings: SourceProductBaseCode=PW,SS,VE
  Convective Heat Transfer : fl_lib/Thermal/Thermal Elements/Convective Heat Transfer  area=1e-4 m^2  heat_tr_coeff=20 W/(K*m^2)  T_specify=off  T_priority=None  T=0 K  T_nominal_specify=off  T_nominal_unit=K  T_nominal_value=1  Q_specify=off  Q_priority=None  Q=0 W  Q_nominal_specify=off  Q_nominal_unit=W  Q_nominal_value=1
      settings: SourceProductBaseCode=PW,SS,VE
  Data Store Write : DataStoreWrite  DataStoreName=C  IndexOptions=Index vector (dialog)  Indices=1  OutputSizes=1
  PS-Simulink Converter : nesl_utility/PS-Simulink Converter  PhysicalDomain=network_engine_domain  SubClassName=ps_output  LeftPortType=input  RightPortType=output  PseudoPeriodic=off  Frequencies=[]  VectorFormat=inherit  Unit=inherit  AffineConversion=off
      settings: SourceProductBaseCode=SS,PW,VE
  Scope : Scope
  Temperature Sensor : fl_lib/Thermal/Thermal Sensors/Temperature Sensor
      settings: SourceProductBaseCode=PW,SS,VE
  Thermal Mass : fl_lib/Thermal/Thermal Elements/Thermal Mass  mass=1 kg  sp_heat=447 J/(K*kg)  T_specify=off  T_priority=High  T=300 K  T_nominal_specify=off  T_nominal_unit=K  T_nominal_value=1  Q_specify=off  Q_priority=None  Q=0 W  Q_nominal_specify=off  Q_nominal_unit=W  Q_nominal_value=1
      settings: SourceProductBaseCode=PW,SS,VE
  Thermal Reference : fl_lib/Thermal/Thermal Elements/Thermal Reference
      settings: SourceProductBaseCode=PW,SS,VE
  Connection Port : PMIOPort  Side=Left
  wires:
  PS-Simulink Converter/1 -> Data Store Write/1, Scope/1
  connections:
  Connection Port/RConn1 -- Conductive Heat Transfer/LConn1
  Thermal Mass/LConn1 -- Conductive Heat Transfer/RConn1 -- Convective Heat Transfer/LConn1
  Temperature Sensor/LConn1 -- Convective Heat Transfer/RConn1
  Thermal Reference/LConn1 -- Temperature Sensor/RConn1
  PS-Simulink Converter/LConn1 -- Temperature Sensor/RConn2

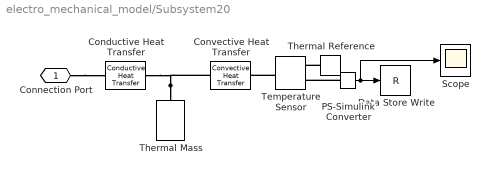
== system electro_mechanical_model/Subsystem20 ==
  Conductive Heat Transfer : fl_lib/Thermal/Thermal Elements/Conductive Heat Transfer  area=1e-4 m^2  thickness=0.1 m  th_cond=401 W/(K*m)  T_specify=off  T_priority=None  T=0 K  T_nominal_specify=off  T_nominal_unit=K  T_nominal_value=1  Q_specify=off  Q_priority=None  Q=0 W  Q_nominal_specify=off  Q_nominal_unit=W  Q_nominal_value=1
      settings: SourceProductBaseCode=PW,SS,VE
  Convective Heat Transfer : fl_lib/Thermal/Thermal Elements/Convective Heat Transfer  area=1e-4 m^2  heat_tr_coeff=20 W/(K*m^2)  T_specify=off  T_priority=None  T=0 K  T_nominal_specify=off  T_nominal_unit=K  T_nominal_value=1  Q_specify=off  Q_priority=None  Q=0 W  Q_nominal_specify=off  Q_nominal_unit=W  Q_nominal_value=1
      settings: SourceProductBaseCode=PW,SS,VE
  Data Store Write : DataStoreWrite  DataStoreName=R  IndexOptions=Index vector (dialog)  Indices=1  OutputSizes=1
  PS-Simulink Converter : nesl_utility/PS-Simulink Converter  PhysicalDomain=network_engine_domain  SubClassName=ps_output  LeftPortType=input  RightPortType=output  PseudoPeriodic=off  Frequencies=[]  VectorFormat=inherit  Unit=inherit  AffineConversion=off
      settings: SourceProductBaseCode=SS,PW,VE
  Scope : Scope
  Temperature Sensor : fl_lib/Thermal/Thermal Sensors/Temperature Sensor
      settings: SourceProductBaseCode=PW,SS,VE
  Thermal Mass : fl_lib/Thermal/Thermal Elements/Thermal Mass  mass=1 kg  sp_heat=447 J/(K*kg)  T_specify=off  T_priority=High  T=300 K  T_nominal_specify=off  T_nominal_unit=K  T_nominal_value=1  Q_specify=off  Q_priority=None  Q=0 W  Q_nominal_specify=off  Q_nominal_unit=W  Q_nominal_value=1
      settings: SourceProductBaseCode=PW,SS,VE
  Thermal Reference : fl_lib/Thermal/Thermal Elements/Thermal Reference
      settings: SourceProductBaseCode=PW,SS,VE
  Connection Port : PMIOPort  Side=Left
  wires:
  PS-Simulink Converter/1 -> Data Store Write/1, Scope/1
  connections:
  Connection Port/RConn1 -- Conductive Heat Transfer/LConn1
  Thermal Mass/LConn1 -- Conductive Heat Transfer/RConn1 -- Convective Heat Transfer/LConn1
  Temperature Sensor/LConn1 -- Convective Heat Transfer/RConn1
  Thermal Reference/LConn1 -- Temperature Sensor/RConn1
  PS-Simulink Converter/LConn1 -- Temperature Sensor/RConn2

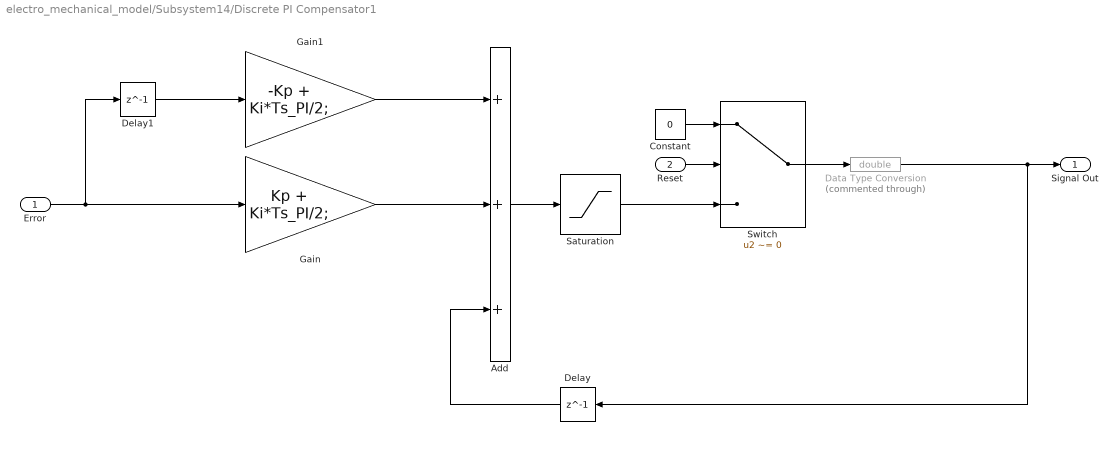
== system electro_mechanical_model/Subsystem14/Discrete PI Compensator1 ==
  Error : Inport
  Reset : Inport  Port=2
  Add : Sum  Inputs=+++  AccumDataTypeStr=single
  Constant : Constant  Value=0
  Data Type Conversion : DataTypeConversion  Commented=through  OutDataTypeStr=double  SaturateOnIntegerOverflow=off  RndMeth=Floor
  Delay : Delay  DelayLength=1
  Delay1 : Delay  DelayLength=1  InitialCondition=Initial_Condition
  Gain : Gain  Gain=Kp + Ki*Ts_PI/2;
  Gain1 : Gain  Gain="-Kp +  Ki*Ts_PI/2;"
  Saturation : Saturate  UpperLimit=UpSat  LowerLimit=LowSat  OutDataTypeStr=single
  Switch : Switch  Criteria=u2 ~= 0  Threshold=0.5  SaturateOnIntegerOverflow=off  InputSameDT=off
  Signal Out : Outport
  wires:
  Data Type Conversion/1 -> Signal Out/1, Delay/1
  Constant/1 -> Switch/1
  Switch/1 -> Data Type Conversion/1
  Reset/1 -> Switch/2
  Saturation/1 -> Switch/3
  Gain1/1 -> Add/1
  Delay1/1 -> Gain1/1
  Gain/1 -> Add/2
  Delay/1 -> Add/3
  Error/1 -> Gain/1, Delay1/1
  Add/1 -> Saturation/1

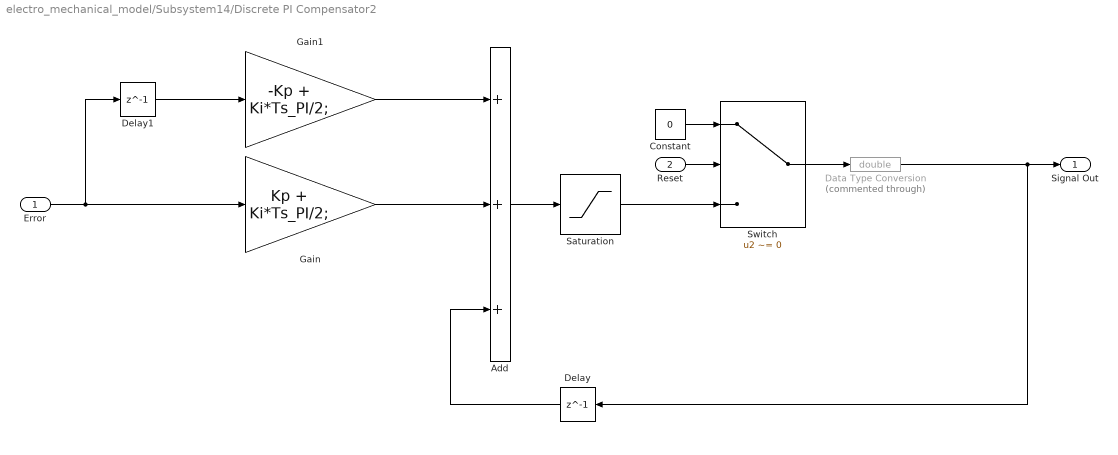
== system electro_mechanical_model/Subsystem14/Discrete PI Compensator2 ==
  Error : Inport
  Reset : Inport  Port=2
  Add : Sum  Inputs=+++  AccumDataTypeStr=single
  Constant : Constant  Value=0
  Data Type Conversion : DataTypeConversion  Commented=through  OutDataTypeStr=double  SaturateOnIntegerOverflow=off  RndMeth=Floor
  Delay : Delay  DelayLength=1
  Delay1 : Delay  DelayLength=1  InitialCondition=Initial_Condition
  Gain : Gain  Gain=Kp + Ki*Ts_PI/2;
  Gain1 : Gain  Gain="-Kp +  Ki*Ts_PI/2;"
  Saturation : Saturate  UpperLimit=UpSat  LowerLimit=LowSat  OutDataTypeStr=single
  Switch : Switch  Criteria=u2 ~= 0  Threshold=0.5  SaturateOnIntegerOverflow=off  InputSameDT=off
  Signal Out : Outport
  wires:
  Add/1 -> Saturation/1
  Error/1 -> Delay1/1, Gain/1
  Delay/1 -> Add/3
  Gain/1 -> Add/2
  Delay1/1 -> Gain1/1
  Gain1/1 -> Add/1
  Saturation/1 -> Switch/3
  Reset/1 -> Switch/2
  Switch/1 -> Data Type Conversion/1
  Constant/1 -> Switch/1
  Data Type Conversion/1 -> Delay/1, Signal Out/1
